simulink model "asbdhc2_FlyAirliner"  (R2024b)
settings: Solver=ode23  StartTime=0.0  StopTime=Inf  MaxStep=1/30  RelTol=1e-2  AbsTol=1e-3  EnableMultiTasking=on
PreLoadFcn:
  | load asbdhc2_init;
values from neighbouring files (symbols this model uses):
  beaver_b = 14.63    [AircraftParam.mat]
  beaver_c = 1.5875    [AircraftParam.mat]
  beaver_init_p = 0    [AircraftParam.mat]
  beaver_init_pitch = 0.13029612885    [AircraftParam.mat]
  beaver_init_q = 0    [AircraftParam.mat]
  beaver_init_r = 0    [AircraftParam.mat]
  beaver_init_roll = 0    [AircraftParam.mat]
  beaver_mass = 2288.231    [AircraftParam.mat]
  Cl0 = 0.000591    [AircraftParam.mat]
  Cl_alpha2_dpt = -0.01406    [AircraftParam.mat]
  Cl_beta = -0.0618    [AircraftParam.mat]
  Cl_da = -0.09917    [AircraftParam.mat]
  Cl_da_alpha = -0.08269    [AircraftParam.mat]
  Cl_dr = 0.006934    [AircraftParam.mat]
  Cl_p = -0.5045    [AircraftParam.mat]
  Cl_r = 0.1695    [AircraftParam.mat]
  Cm0 = 0.09448    [AircraftParam.mat]
  Cm_alpha = -0.6028    [AircraftParam.mat]
  Cm_alpha2 = -2.14    [AircraftParam.mat]
  Cm_beta2 = 0.6921    [AircraftParam.mat]
  Cm_de = -1.921    [AircraftParam.mat]
  Cm_df = 0.4072    [AircraftParam.mat]
  Cm_dpt = -0.07895    [AircraftParam.mat]
  Cm_q = -15.56    [AircraftParam.mat]
  Cm_r = -0.3118    [AircraftParam.mat]
  Cn0 = -0.003117    [AircraftParam.mat]
  Cn_beta = 0.006719    [AircraftParam.mat]
  Cn_beta3 = 0.1373    [AircraftParam.mat]
  Cn_da = -0.003872    [AircraftParam.mat]
  Cn_dpt3 = -0.003026    [AircraftParam.mat]
  Cn_dr = -0.08265    [AircraftParam.mat]
  Cn_p = -0.1585    [AircraftParam.mat]
  Cn_q = 0.1595    [AircraftParam.mat]
  Cn_r = -0.1112    [AircraftParam.mat]
  Cx0 = -0.03554    [AircraftParam.mat]
  Cx_alpha = 0.00292    [AircraftParam.mat]
  Cx_alpha2 = 5.459    [AircraftParam.mat]
  Cx_alpha3 = -5.162    [AircraftParam.mat]
  Cx_df = -0.09447    [AircraftParam.mat]
  Cx_df_alpha = 1.106    [AircraftParam.mat]
  Cx_dpt = 0.1161    [AircraftParam.mat]
  Cx_dpt2_alpha = 0.1453    [AircraftParam.mat]
  Cx_dr = 0.03412    [AircraftParam.mat]
  Cx_q = -0.6748    [AircraftParam.mat]
  Cy0 = -0.002226    [AircraftParam.mat]
  Cy_beta = -0.7678    [AircraftParam.mat]
  Cy_da = -0.02956    [AircraftParam.mat]
  Cy_dr = 0.1158    [AircraftParam.mat]
  Cy_dr_alpha = 0.5238    [AircraftParam.mat]
  Cy_p = -0.124    [AircraftParam.mat]
  Cy_r = 0.3666    [AircraftParam.mat]
  Cz0 = -0.05504    [AircraftParam.mat]
  Cz_alpha = -5.578    [AircraftParam.mat]
  Cz_alpha3 = 3.442    [AircraftParam.mat]
  Cz_de = -0.398    [AircraftParam.mat]
  Cz_de_beta = -15.93    [AircraftParam.mat]
  Cz_df = -1.377    [AircraftParam.mat]
  Cz_df_alpha = -1.261    [AircraftParam.mat]
  Cz_dpt = -0.1563    [AircraftParam.mat]
  Cz_q = -2.988    [AircraftParam.mat]
  heading0 = 0    [AircraftParam.mat]
  uaero0 = [-0.0317656979071 -0.0320210159663 -0.0365180369264 0]    [AircraftParam.mat]
  xme_0 = [3000 0 -50]    [AircraftParam.mat]
undefined symbols (not defined in the file or in its folder): F, Light, MIL
libraries: aerolibsim3d x4, aerolibwind2 x3, aerolibasang x2, simulink x2, aerolibconvert2 x2, shared6dof x1, aerolibadyn x1, aerolibatmos2 x1, cstblocks x1, aerolibanimutils x1, sim3dlib x1
(part 2 of 2)

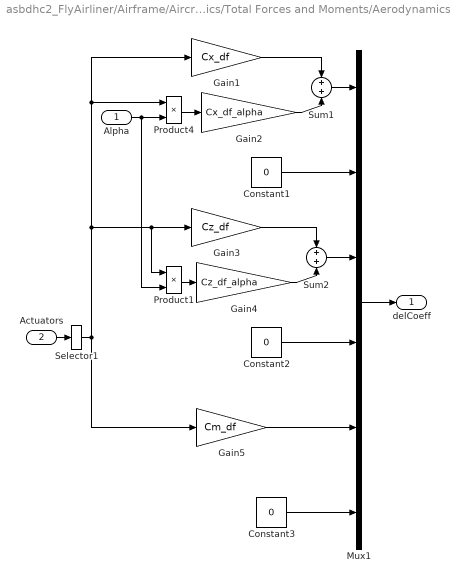
== system asbdhc2_FlyAirliner/Airframe/Aircraft Dynamics/Total Forces and Moments/Aerodynamics/Actuator Increments/Flap ==
  Alpha : Inport  Unit=rad
  Actuators : Inport  Port=2  Unit=rad
  Constant1 : Constant  Value=0
  Constant2 : Constant  Value=0
  Constant3 : Constant  Value=0
  Gain1 : Gain  Gain=Cx_df  SaturateOnIntegerOverflow=on  OutDataTypeStr=Inherit: Same as input  ParamDataTypeStr=Inherit: Same as input
  Gain2 : Gain  Gain=Cx_df_alpha  SaturateOnIntegerOverflow=on  OutDataTypeStr=Inherit: Same as input  ParamDataTypeStr=Inherit: Same as input
  Gain3 : Gain  Gain=Cz_df  SaturateOnIntegerOverflow=on  OutDataTypeStr=Inherit: Same as input  ParamDataTypeStr=Inherit: Same as input
  Gain4 : Gain  Gain=Cz_df_alpha  SaturateOnIntegerOverflow=on  OutDataTypeStr=Inherit: Same as input  ParamDataTypeStr=Inherit: Same as input
  Gain5 : Gain  Gain=Cm_df  SaturateOnIntegerOverflow=on  OutDataTypeStr=Inherit: Same as input  ParamDataTypeStr=Inherit: Same as input
  Mux1 : Mux  Inputs=6
  Product1 : Product  InputSameDT=on  SaturateOnIntegerOverflow=on  OutDataTypeStr=Inherit: Same as first input
  Product4 : Product  InputSameDT=on  SaturateOnIntegerOverflow=on  OutDataTypeStr=Inherit: Same as first input
  Selector1 : Selector  IndexMode=Zero-based  InputPortWidth=4  IndexOptions=Index vector (dialog)  Indices=3  OutputSizes=1
  Sum1 : Sum  SaturateOnIntegerOverflow=on
  Sum2 : Sum  SaturateOnIntegerOverflow=on
  delCoeff : Outport  VectorParamsAs1DForOutWhenUnconnected=off
  wires:
  Selector1/1 -> Gain1/1, Product4/1, Product1/1, Gain3/1, Gain5/1
  Actuators/1 -> Selector1/1
  Gain5/1 -> Mux1/5
  Gain3/1 -> Sum2/1
  Gain4/1 -> Sum2/2
  Product1/1 -> Gain4/1
  Gain1/1 -> Sum1/1
  Gain2/1 -> Sum1/2
  Product4/1 -> Gain2/1
  Alpha/1 -> Product1/2, Product4/2
  Mux1/1 -> delCoeff/1
  Sum1/1 -> Mux1/1
  Sum2/1 -> Mux1/3
  Constant1/1 -> Mux1/2
  Constant2/1 -> Mux1/4
  Constant3/1 -> Mux1/6

== system asbdhc2_FlyAirliner/Airframe/Aircraft Dynamics/Total Forces and Moments/Aerodynamics/Actuator Increments/Rudder ==
  Alpha : Inport  Unit=rad
  Actuators : Inport  Port=2  Unit=rad
  Constant1 : Constant  Value=0
  Constant2 : Constant  Value=0
  Gain1 : Gain  Gain=Cl_dr  SaturateOnIntegerOverflow=on  OutDataTypeStr=Inherit: Same as input  ParamDataTypeStr=Inherit: Same as input
  Gain2 : Gain  Gain=Cn_dr  SaturateOnIntegerOverflow=on  OutDataTypeStr=Inherit: Same as input  ParamDataTypeStr=Inherit: Same as input
  Gain3 : Gain  Gain=Cy_dr_alpha  SaturateOnIntegerOverflow=on  OutDataTypeStr=Inherit: Same as input  ParamDataTypeStr=Inherit: Same as input
  Gain4 : Gain  Gain=Cy_dr  SaturateOnIntegerOverflow=on  OutDataTypeStr=Inherit: Same as input  ParamDataTypeStr=Inherit: Same as input
  Gain5 : Gain  Gain=Cx_dr  SaturateOnIntegerOverflow=on  OutDataTypeStr=Inherit: Same as input  ParamDataTypeStr=Inherit: Same as input
  Mux1 : Mux  Inputs=6
  Product1 : Product  InputSameDT=on  SaturateOnIntegerOverflow=on  OutDataTypeStr=Inherit: Same as first input
  Selector1 : Selector  IndexMode=Zero-based  InputPortWidth=4  IndexOptions=Index vector (dialog)  Indices=2  OutputSizes=1
  Sum1 : Sum  SaturateOnIntegerOverflow=on
  delCoeff : Outport  VectorParamsAs1DForOutWhenUnconnected=off
  wires:
  Gain5/1 -> Mux1/1
  Gain4/1 -> Sum1/1
  Gain3/1 -> Sum1/2
  Gain1/1 -> Mux1/4
  Gain2/1 -> Mux1/6
  Product1/1 -> Gain3/1
  Alpha/1 -> Product1/2
  Mux1/1 -> delCoeff/1
  Actuators/1 -> Selector1/1
  Sum1/1 -> Mux1/2
  Constant1/1 -> Mux1/3
  Constant2/1 -> Mux1/5
  Selector1/1 -> Gain5/1, Gain4/1, Product1/1, Gain1/1, Gain2/1

== system asbdhc2_FlyAirliner/Airframe/Aircraft Dynamics/Total Forces and Moments/Aerodynamics/Body Rate Damping/p ==
  Constant1 : Constant  Value=0
  Constant2 : Constant  Value=Cy_p
  Constant3 : Constant  Value=Cl_p
  Constant4 : Constant  Value=Cn_p
  Mux1 : Mux  Inputs=6
  delCoeff : Outport  VectorParamsAs1DForOutWhenUnconnected=off
  wires:
  Constant2/1 -> Mux1/2
  Mux1/1 -> delCoeff/1
  Constant1/1 -> Mux1/5, Mux1/3, Mux1/1
  Constant4/1 -> Mux1/6
  Constant3/1 -> Mux1/4

== system asbdhc2_FlyAirliner/Airframe/Aircraft Dynamics/Total Forces and Moments/Aerodynamics/Body Rate Damping/q ==
  Constant1 : Constant  Value=0
  Constant2 : Constant  Value=Cz_q
  Constant3 : Constant  Value=Cx_q
  Constant4 : Constant  Value=Cm_q
  Constant5 : Constant  Value=Cn_q
  Mux1 : Mux  Inputs=6
  delCoeff : Outport  VectorParamsAs1DForOutWhenUnconnected=off
  wires:
  Constant2/1 -> Mux1/3
  Constant5/1 -> Mux1/6
  Constant1/1 -> Mux1/4, Mux1/2
  Constant4/1 -> Mux1/5
  Constant3/1 -> Mux1/1
  Mux1/1 -> delCoeff/1

== system asbdhc2_FlyAirliner/Airframe/Aircraft Dynamics/Total Forces and Moments/Aerodynamics/Body Rate Damping/r ==
  Constant : Constant  Value=0
  Constant1 : Constant  Value=Cy_r
  Constant2 : Constant  Value=Cl_r
  Constant3 : Constant  Value=Cm_r
  Constant4 : Constant  Value=Cn_r
  Mux1 : Mux  Inputs=6
  delCoeff : Outport  VectorParamsAs1DForOutWhenUnconnected=off
  wires:
  Constant3/1 -> Mux1/5
  Constant1/1 -> Mux1/2
  Constant4/1 -> Mux1/6
  Constant2/1 -> Mux1/4
  Constant/1 -> Mux1/3, Mux1/1
  Mux1/1 -> delCoeff/1
